simulink model "Mat"  (R2017b)
settings: Solver=VariableStepAuto  StartTime=0.0  StopTime=10.0  RelTol=1e-3
settings Model: Creator=ng8a07e  LastModifiedBy=ng8a07e

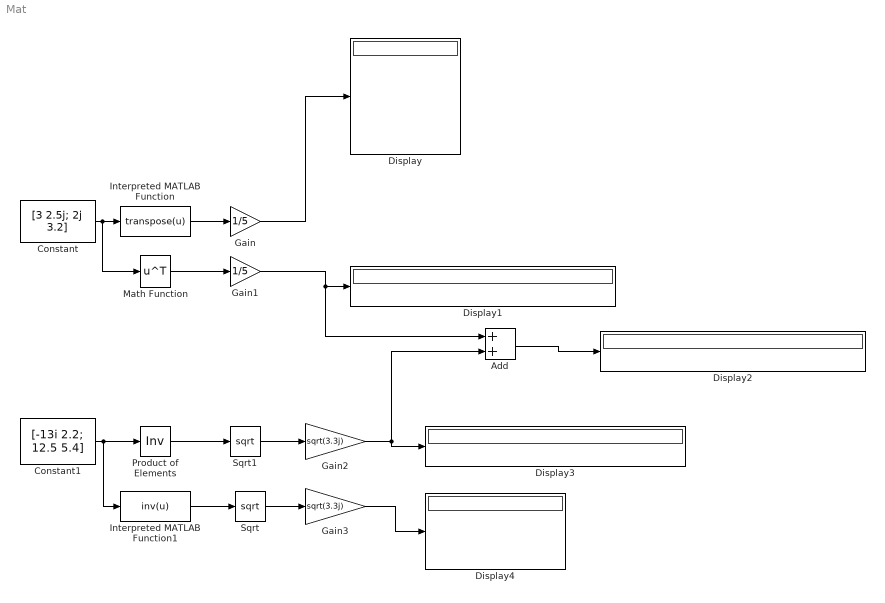
== system Mat ==
  Add : Sum
  Constant : Constant  Value=[3 2.5j; 2j 3.2]
  Constant1 : Constant  Value=[-13i 2.2; 12.5 5.4]
  Display{,1..4} (5 alike) : Display
  Gain : Gain  Gain=1/5
  Gain1 : Gain  Gain=1/5
  Gain2 : Gain  Gain=sqrt(3.3j)
  Gain3 : Gain  Gain=sqrt(3.3j)
  Interpreted MATLAB Function : MATLABFcn  MATLABFcn=transpose(u)
  Interpreted MATLAB Function1 : MATLABFcn  MATLABFcn=inv(u)
  Math Function : Math  Operator=transpose  SaturateOnIntegerOverflow=on
  Product of Elements : Product  Inputs=/  Multiplication=Matrix(*)
  Sqrt : Sqrt  SaturateOnIntegerOverflow=on
  Sqrt1 : Sqrt  SaturateOnIntegerOverflow=on
  wires:
  Constant/1 -> Math Function/1, Interpreted MATLAB Function/1
  Interpreted MATLAB Function/1 -> Gain/1
  Math Function/1 -> Gain1/1
  Interpreted MATLAB Function1/1 -> Sqrt/1
  Constant1/1 -> Interpreted MATLAB Function1/1, Product of Elements/1
  Product of Elements/1 -> Sqrt1/1
  Sqrt1/1 -> Gain2/1
  Sqrt/1 -> Gain3/1
  Gain/1 -> Display/1
  Gain1/1 -> Add/1, Display1/1
  Add/1 -> Display2/1
  Gain2/1 -> Add/2, Display3/1
  Gain3/1 -> Display4/1
